simulink model "FullModel"  (R2021b)
settings: Solver=FixedStepAuto  StartTime=0.0  StopTime=10.0  FixedStep=10  RelTol=1e-3
values from neighbouring files (symbols this model uses):
  Model_input = C(Samplenumber,:)    [geting_input_to_FullModel.m]
settings Model: Creator=Admin  LastModifiedBy=Admin

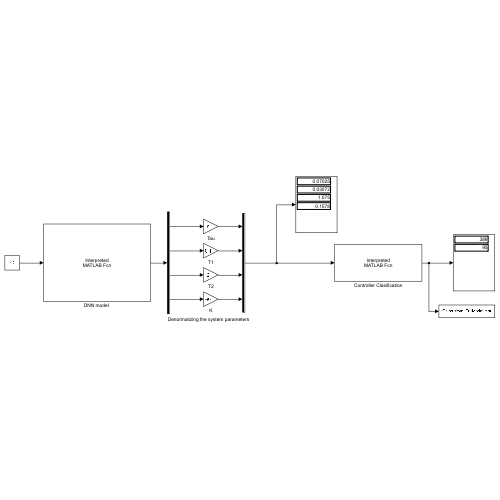
[thumbnail: Simulink's stored preview of the top-level diagram]
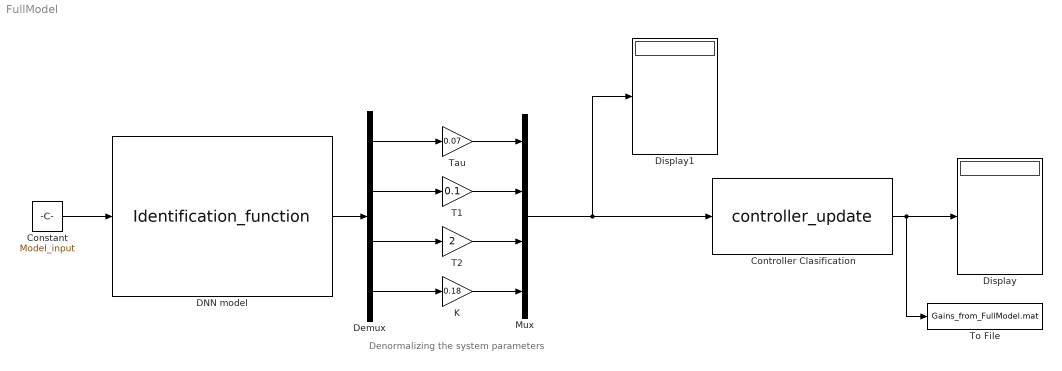
== system FullModel ==
  note: Denormalizing the system parameters
  Constant : Constant  Value=Model_input
  Controller Clasification : MATLABFcn  MATLABFcn=controller_update  OutputDimensions=2
  "DNN model " : MATLABFcn  MATLABFcn=Identification_function  OutputDimensions=4
  Demux : Demux
  Display : Display
  Display1 : Display
  K : Gain  Gain=0.18
  Mux : Mux
  T1 : Gain  Gain=0.1
  T2 : Gain  Gain=2
  Tau : Gain  Gain=0.07
  To File : ToFile  Filename=Gains_from_FullModel.mat  MatrixName=KPandKD
  wires:
  Constant/1 -> "DNN model "/1
  "DNN model "/1 -> Demux/1
  Demux/1 -> Tau/1
  Demux/2 -> T1/1
  Demux/3 -> T2/1
  Demux/4 -> K/1
  T1/1 -> Mux/2
  Tau/1 -> Mux/1
  T2/1 -> Mux/3
  K/1 -> Mux/4
  Controller Clasification/1 -> To File/1, Display/1
  Mux/1 -> Display1/1, Controller Clasification/1
